simulink model "low_pass_simulink"  (R2016b)
settings: Solver=VariableStepAuto  StartTime=0.0  StopTime=50  RelTol=1e-3
libraries: simulink x1
settings Model: Creator=u18b15  LastModifiedBy=u18b15

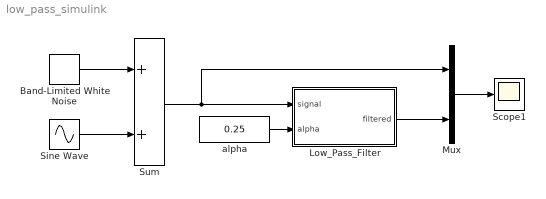
== system low_pass_simulink ==
  Band-Limited White Noise : simulink/Sources/Band-Limited White Noise  Cov=[0.01]  Ts=0.1  seed=[23341]
  Low_Pass_Filter : Subsystem
  Mux : Mux  Inputs=2
  Scope1 : Scope
  Sine Wave : Sin  Amplitude=4  SampleTime=0
  Sum : Sum
  alpha : Constant  Value=0.25
  wires:
  Band-Limited White Noise/1 -> Sum/1
  Sine Wave/1 -> Sum/2
  Mux/1 -> Scope1/1
  Sum/1 -> Mux/1, Low_Pass_Filter/1(signal)
  Low_Pass_Filter/1(filtered) -> Mux/2
  alpha/1 -> Low_Pass_Filter/2(alpha)

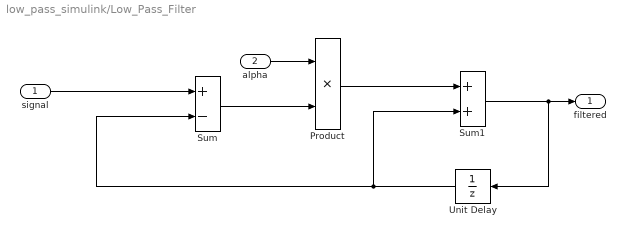
== system low_pass_simulink/Low_Pass_Filter ==
  signal : Inport
  alpha : Inport  Port=2
  Product : Product
  Sum : Sum  Inputs=+-
  Sum1 : Sum
  Unit Delay : UnitDelay  SampleTime=-1
  filtered : Outport
  wires:
  alpha/1 -> Product/1
  signal/1 -> Sum/1
  Sum/1 -> Product/2
  Product/1 -> Sum1/1
  Sum1/1 -> Unit Delay/1, filtered/1
  Unit Delay/1 -> Sum/2, Sum1/2
